simulink model "tbm_pirelleSnr_ref"  (R2020a)
settings: configuration reference "config_cnv" (kept outside this file)
PreLoadFcn:
  | defParm_cu_tbm_spt
libraries: lib_tbm_presToTbFlag_whl x4, lib_decmp_Calib_pirelle_presSnr_x8 x1
settings Model: Creator=Administrator  LastModifiedBy=bowen.zheng
settings ConfigSetRef: SourceName=config_cnv  SourceLocation=Base Workspace

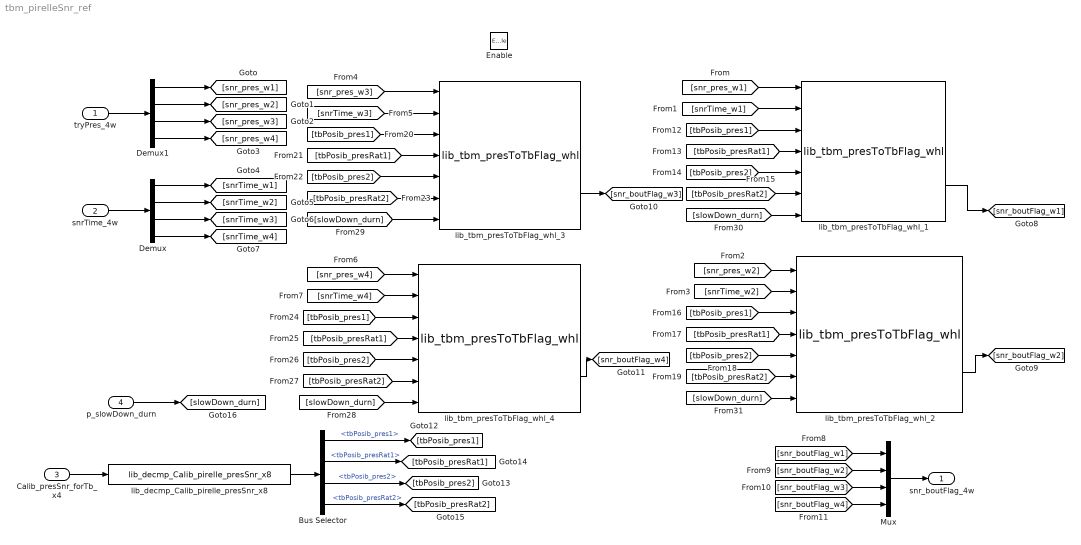
== system tbm_pirelleSnr_ref ==
  tryPres_4w : Inport
  snrTime_4w : Inport  Port=2
  Calib_presSnr_forTb_x4 : Inport  Port=3  OutDataTypeStr=single  PortDimensions=8
  p_slowDown_durn : Inport  Port=4
  Enable : EnablePort  OutDataTypeStr=boolean
  Bus Selector : BusSelector  OutputSignals=tbPosib_pres1,tbPosib_presRat1,tbPosib_pres2,tbPosib_presRat2
  Demux : Demux
  Demux1 : Demux
  Mux : Mux
  lib_decmp_Calib_pirelle_presSnr_x8 : lib_decmp_Calib_pirelle_presSnr_x8/lib_decmp_Calib_pirelle_presSnr_x8  SystemSampleTime=-1  Latency=0  AutoFrameSizeCalculation=off
  lib_tbm_presToTbFlag_whl_{1..4} (4 alike) : lib_tbm_presToTbFlag_whl/lib_tbm_presToTbFlag_whl  SystemSampleTime=-1  Latency=0  AutoFrameSizeCalculation=off
  " snr_boutFlag_4w" : Outport
  wires:
  [snr_boutFlag_w4] -> Mux/4
  [snr_pres_w3] -> lib_tbm_presToTbFlag_whl_3/1
  lib_tbm_presToTbFlag_whl_3/2 -> [snr_boutFlag_w3]
  lib_tbm_presToTbFlag_whl_4/2 -> [snr_boutFlag_w4]
  Bus Selector/1 -> [tbPosib_pres1]  "<tbPosib_pres1>"
  [snr_boutFlag_w3] -> Mux/3
  Demux1/4 -> [snr_pres_w4]
  lib_tbm_presToTbFlag_whl_1/2 -> [snr_boutFlag_w1]
  [tbPosib_pres2] -> lib_tbm_presToTbFlag_whl_1/5
  Demux1/2 -> [snr_pres_w2]
  [snrTime_w3] -> lib_tbm_presToTbFlag_whl_3/2
  [tbPosib_presRat2] -> lib_tbm_presToTbFlag_whl_1/6
  Bus Selector/3 -> [tbPosib_pres2]  "<tbPosib_pres2>"
  Demux/4 -> [snrTime_w4]
  Demux/3 -> [snrTime_w3]
  Bus Selector/4 -> [tbPosib_presRat2]  "<tbPosib_presRat2>"
  Calib_presSnr_forTb_x4/1 -> lib_decmp_Calib_pirelle_presSnr_x8/1
  Demux1/3 -> [snr_pres_w3]
  Demux1/1 -> [snr_pres_w1]
  lib_decmp_Calib_pirelle_presSnr_x8/1 -> Bus Selector/1
  Demux/2 -> [snrTime_w2]
  [tbPosib_presRat1] -> lib_tbm_presToTbFlag_whl_3/4
  [tbPosib_presRat2] -> lib_tbm_presToTbFlag_whl_4/6
  [tbPosib_presRat2] -> lib_tbm_presToTbFlag_whl_3/6
  [snr_boutFlag_w2] -> Mux/2
  [tbPosib_pres2] -> lib_tbm_presToTbFlag_whl_4/5
  snrTime_4w/1 -> Demux/1
  lib_tbm_presToTbFlag_whl_2/2 -> [snr_boutFlag_w2]
  [snr_pres_w1] -> lib_tbm_presToTbFlag_whl_1/1
  [snr_boutFlag_w1] -> Mux/1
  [tbPosib_pres1] -> lib_tbm_presToTbFlag_whl_1/3
  [tbPosib_pres1] -> lib_tbm_presToTbFlag_whl_4/3
  [snrTime_w2] -> lib_tbm_presToTbFlag_whl_2/2
  [tbPosib_presRat1] -> lib_tbm_presToTbFlag_whl_1/4
  tryPres_4w/1 -> Demux1/1
  [tbPosib_pres2] -> lib_tbm_presToTbFlag_whl_3/5
  Demux/1 -> [snrTime_w1]
  [tbPosib_pres2] -> lib_tbm_presToTbFlag_whl_2/5
  [snrTime_w1] -> lib_tbm_presToTbFlag_whl_1/2
  [snrTime_w4] -> lib_tbm_presToTbFlag_whl_4/2
  [tbPosib_pres1] -> lib_tbm_presToTbFlag_whl_3/3
  [tbPosib_presRat1] -> lib_tbm_presToTbFlag_whl_2/4
  Bus Selector/2 -> [tbPosib_presRat1]  "<tbPosib_presRat1>"
  [snr_pres_w4] -> lib_tbm_presToTbFlag_whl_4/1
  [tbPosib_presRat1] -> lib_tbm_presToTbFlag_whl_4/4
  [snr_pres_w2] -> lib_tbm_presToTbFlag_whl_2/1
  Mux/1 -> " snr_boutFlag_4w"/1
  [tbPosib_presRat2] -> lib_tbm_presToTbFlag_whl_2/6
  [tbPosib_pres1] -> lib_tbm_presToTbFlag_whl_2/3
  p_slowDown_durn/1 -> [slowDown_durn]
  [slowDown_durn] -> lib_tbm_presToTbFlag_whl_4/7
  [slowDown_durn] -> lib_tbm_presToTbFlag_whl_3/7
  [slowDown_durn] -> lib_tbm_presToTbFlag_whl_1/7
  [slowDown_durn] -> lib_tbm_presToTbFlag_whl_2/7
